simulink model "pfb_fir"  (Simulink 7.0)
settings: Solver=FixedStepDiscrete  SolverMode=SingleTasking  StartTime=0.0  StopTime=10.0  RelTol=1e-3
undefined symbols (not defined in the file): pfb_coefs
libraries: xbsIndex_r4 x385
(part 1 of 27)
settings Model: Creator=homin  LastModifiedBy=homin
settings DebuggingCC: SaveWithParameterizedLinksMsg=none  SignalResolutionControl=TryResolveAllWithWarning  MultiTaskDSMMsg=warning  MultiTaskCondExecSysMsg=none  StrictBusMsg=None
settings RTWCC: IncludeERTFirstTime=on
settings GRTTargetCC: TargetFcnLib=ansi_tfl_tmw.mat

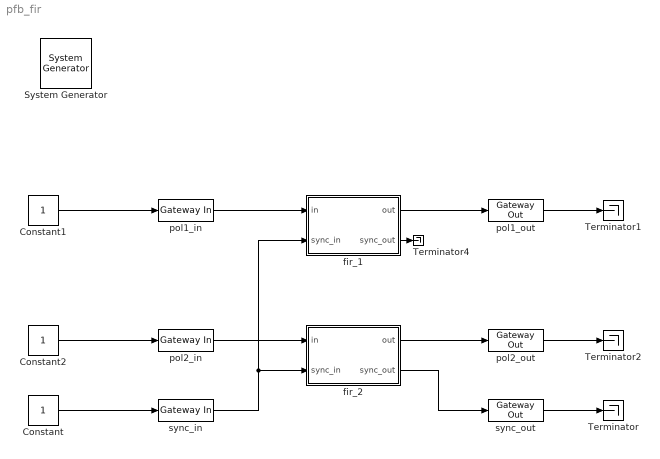
== system pfb_fir ==
  " System Generator" : xbsIndex_r4/ System Generator  Tag=genX  SystemSampleTime=-1  xilinxfamily=Virtex2P  part=xc2vp40  speed=-6  package=ff1152  synthesis_tool=XST  clock_wrapper=Clock Enables  directory=./pfb_fir_core  testbench=off  simulink_period=1  sysclk_period=100  dcm_input_clock_period=100  incr_netlist=off  trim_vbits=Everywhere in SubSystem  dbl_ovrd=According to Block Masks  core_generation=According to Block Masks  run_coregen=off  deprecated_control=off  eval_field=0  block_type=sysgen
      settings: block_version=10.1.3
  Constant : Constant  OutDataType=sfix(16)  OutScaling=2^0
  Constant1 : Constant  OutDataType=sfix(16)  OutScaling=2^0
  Constant2 : Constant  OutDataType=sfix(16)  OutScaling=2^0
  Terminator{,1..2,4} (4 alike) : Terminator
  fir_1 : Subsystem  AncestorBlock=newfft_library/FIR/fir  mask(FIR Filter){coefs=pfb_coefs(1024,6), n_bits_c=9, bin_pt_c=8, n_bits_d=8, bin_pt_d=7, n_bits_o=9, bin_pt_o=7, coef_bram=on, delay_bram=on, mult_latency=3, add_latency=1, show_sbo=on, munge_submasks=DumbDown}
      mask prompts: coefs "Tap Coefficients"; n_bits_c "Number of Coefficient Bits"; bin_pt_c "Coefficient Binary Point"; n_bits_d "Number of Data Bits"; bin_pt_d "Data Binary Point"; n_bits_o "Number of Bits Out"; bin_pt_o "Binary Point Out"; coef_bram "Use BRAM for Coefficients"; delay_bram "Use BRAM for Delay"; mult_latency "Multiplier Latency"; add_latency "Adder Latency"; show_sbo "Show Sub-Block Options"; munge_submasks "Sub-Block Masks"
      mask help: A Finite Impluse Response Filter. This FIR filter does not have provisions for folding the input sequence to improve multiplier efficiency, so it is suboptimal for "regular" (i.e. non-WOLA) FIR filters. It is intended primarily for WOLA (Weighted OverLap Add) FIR filters.
      mask init:
      | tic
      | fir_init(gcb, ...
      |   coefs, ...
      |   n_bits_c, ...
      |   bin_pt_c, ...
      |   n_bits_d, ...
      |   bin_pt_d, ...
      |   n_bits_o, ...
      |   bin_pt_o, ...
      |   coef_bram, ...
      |   delay_bram, ...
      |   mult_latency, ...
      |   add_latency, ...
      |   lower(get_param(gcb,'munge_submasks')) );
      | disp('fir_init complete.');
      | toc
      settings: AttributesFormatString=|
      | 6 taps
      | 9_8 coefs
      | 8_7 in
      | 9_7 out
      mask Help:
      | <pre>
      | Description::
      | 
      | A Finite Impluse Response Filter.
      | 
      | This Finite Impluse Response Filter does not have provisions for folding the input
      | sequence to improve multiplier efficiency, so it is suboptimal for "regular" (i.e. non-WOLA)
      | FIR filters.  It is intended primarily for WOLA (Weighted OverLap Add) FIR filters.
      | 
      | Mask Parameters::
      | 
      | Coefficiant(s) (coefs): Matrix of real double(s) to use as coefficient(s).
      | One column per tap.  Multiple rows will create a WOLA filter.
      | These should be specified as doubles.  They will be rounded/saturated according to the
      | specified number of bits (n_bits_c) and binary point (bin_pt_c).
      | 
      | Number of Coefficient Bits (n_bits_c): The number of bits used for the fixed point binary
      | representation of the coefficient(s).
      | 
      | Coefficient Binary Point (bin_pt_c): The binary point of the fixed point binary representation
      | of the coefficient(s).
      | 
      | Number of Data Bits (n_bits_d): The number of bits for real/imaginary components of the data.
      | 
      | Data Binary Point (bin_pt_d): The binary point for real/imaginary components of the data.
      | 
      | Number of Bits Out (n_bits_o): Specifies the width of the output (overflow wraps).
      | The internal adders will use a bit width of (n_bits_o-bin_pt_o+bin_pt_c+bin_pt_d).
      | 
      | Binary Point Out (bin_pt_o): Specifies the binary point of the output (quantization truncates).
      | The internal adders will use a binary point of (bin_pt_c+bin_pt_d).
      | 
      | Use BRAM for Coefficients (coef_bram): Check this checkbox to store the coefficients in BRAM.
      | If unchecked, the coefficients will be stored in distributed memory (i.e. slices).
      | This is only relevant is length(coef) is greater than 1; otherwise, a constant block is used.
      | 
      | Use BRAM for Delay (delay_bram): Check this checkbox to implement the delay using BRAM.
      | If unchecked, the delay will be implemented using SLR16 elements (i.e. slices).
      | 
      | Multiplier Latency (mult_latency): Latency to use for the underlying multiplier.
      | 
      | Adder Latency (add_latency): Latency to use for the underlying adder.
      | </pre>
      mask StyleString: edit,edit,edit,edit,edit,edit,edit,checkbox,checkbox,edit,edit,checkbox,popup(Keep|DumbDown|Unmask)
      mask CallbackString:
      | |||||||||||mvs=get_param(gcb,'MaskVisibilityString');
      | if strcmp(get_param(gcb,'show_sbo'),'on')
      |   onoff='on';
      | else
      |   onoff='off';
      | end
      | mvs=regexprep(mvs,'o[nf]*$',onoff);
      | set_param(gcb,'MaskVisibilityString',mvs);
      | |
  fir_2 : Subsystem  AncestorBlock=newfft_library/FIR/fir  mask(FIR Filter){coefs=pfb_coefs(1024,6), n_bits_c=9, bin_pt_c=8, n_bits_d=8, bin_pt_d=7, n_bits_o=9, bin_pt_o=7, coef_bram=on, delay_bram=on, mult_latency=3, add_latency=1, show_sbo=on, munge_submasks=DumbDown}
      mask prompts: coefs "Tap Coefficients"; n_bits_c "Number of Coefficient Bits"; bin_pt_c "Coefficient Binary Point"; n_bits_d "Number of Data Bits"; bin_pt_d "Data Binary Point"; n_bits_o "Number of Bits Out"; bin_pt_o "Binary Point Out"; coef_bram "Use BRAM for Coefficients"; delay_bram "Use BRAM for Delay"; mult_latency "Multiplier Latency"; add_latency "Adder Latency"; show_sbo "Show Sub-Block Options"; munge_submasks "Sub-Block Masks"
      mask help: A Finite Impluse Response Filter. This FIR filter does not have provisions for folding the input sequence to improve multiplier efficiency, so it is suboptimal for "regular" (i.e. non-WOLA) FIR filters. It is intended primarily for WOLA (Weighted OverLap Add) FIR filters.
      mask init: same as pfb_fir/fir_1
      settings: AttributesFormatString=|
      | 6 taps
      | 9_8 coefs
      | 8_7 in
      | 9_7 out
      mask Help:
      | <pre>
      | Description::
      | 
      | A Finite Impluse Response Filter.
      | 
      | This Finite Impluse Response Filter does not have provisions for folding the input
      | sequence to improve multiplier efficiency, so it is suboptimal for "regular" (i.e. non-WOLA)
      | FIR filters.  It is intended primarily for WOLA (Weighted OverLap Add) FIR filters.
      | 
      | Mask Parameters::
      | 
      | Coefficiant(s) (coefs): Matrix of real double(s) to use as coefficient(s).
      | One column per tap.  Multiple rows will create a WOLA filter.
      | These should be specified as doubles.  They will be rounded/saturated according to the
      | specified number of bits (n_bits_c) and binary point (bin_pt_c).
      | 
      | Number of Coefficient Bits (n_bits_c): The number of bits used for the fixed point binary
      | representation of the coefficient(s).
      | 
      | Coefficient Binary Point (bin_pt_c): The binary point of the fixed point binary representation
      | of the coefficient(s).
      | 
      | Number of Data Bits (n_bits_d): The number of bits for real/imaginary components of the data.
      | 
      | Data Binary Point (bin_pt_d): The binary point for real/imaginary components of the data.
      | 
      | Number of Bits Out (n_bits_o): Specifies the width of the output (overflow wraps).
      | The internal adders will use a bit width of (n_bits_o-bin_pt_o+bin_pt_c+bin_pt_d).
      | 
      | Binary Point Out (bin_pt_o): Specifies the binary point of the output (quantization truncates).
      | The internal adders will use a binary point of (bin_pt_c+bin_pt_d).
      | 
      | Use BRAM for Coefficients (coef_bram): Check this checkbox to store the coefficients in BRAM.
      | If unchecked, the coefficients will be stored in distributed memory (i.e. slices).
      | This is only relevant is length(coef) is greater than 1; otherwise, a constant block is used.
      | 
      | Use BRAM for Delay (delay_bram): Check this checkbox to implement the delay using BRAM.
      | If unchecked, the delay will be implemented using SLR16 elements (i.e. slices).
      | 
      | Multiplier Latency (mult_latency): Latency to use for the underlying multiplier.
      | 
      | Adder Latency (add_latency): Latency to use for the underlying adder.
      | </pre>
      mask StyleString: edit,edit,edit,edit,edit,edit,edit,checkbox,checkbox,edit,edit,checkbox,popup(Keep|DumbDown|Unmask)
      mask CallbackString:
      | |||||||||||mvs=get_param(gcb,'MaskVisibilityString');
      | if strcmp(get_param(gcb,'show_sbo'),'on')
      |   onoff='on';
      | else
      |   onoff='off';
      | end
      | mvs=regexprep(mvs,'o[nf]*$',onoff);
      | set_param(gcb,'MaskVisibilityString',mvs);
      | |
  pol1_in : xbsIndex_r4/Gateway In  arith_type=Unsigned  n_bits=16  bin_pt=0  quantization=Truncate  overflow=Wrap  period=1  dbl_ovrd=off  timing_constraint=None  locs_specified=off  LOCs={}  block_type=gatewayin
      settings: infoedit="Gateway in block.  Converts inputs of type Simulink integer, double and fixed point to  Xilinx fixed point type.<P><P>Hardware notes:  In hardware these blocks become top level input ports."  xl_area=[0, 0, 0, 0, 0, 0, 0]  block_version=10.1.3
  pol1_out : xbsIndex_r4/Gateway Out  hdl_port=on  timing_constraint=None  locs_specified=off  LOCs={}  block_type=gatewayout
      settings: infoedit="Gateway out block.  Converts Xilinx fixed point inputs into ouputs of type Simulink integer, double, or fixed point.<P><P>Hardware notes:  In hardware these blocks become top level output ports or are discarded, depending on how they are configured."  xl_area=[0, 0, 0, 0, 0, 0, 0]  block_version=10.1.3
  pol2_in : xbsIndex_r4/Gateway In  arith_type=Unsigned  n_bits=16  bin_pt=0  quantization=Truncate  overflow=Wrap  period=1  dbl_ovrd=off  timing_constraint=None  locs_specified=off  LOCs={}  block_type=gatewayin
      settings: infoedit="Gateway in block.  Converts inputs of type Simulink integer, double and fixed point to  Xilinx fixed point type.<P><P>Hardware notes:  In hardware these blocks become top level input ports."  xl_area=[0, 0, 0, 0, 0, 0, 0]  block_version=10.1.3
  pol2_out : xbsIndex_r4/Gateway Out  hdl_port=on  timing_constraint=None  locs_specified=off  LOCs={}  block_type=gatewayout
      settings: infoedit="Gateway out block.  Converts Xilinx fixed point inputs into ouputs of type Simulink integer, double, or fixed point.<P><P>Hardware notes:  In hardware these blocks become top level output ports or are discarded, depending on how they are configured."  xl_area=[0, 0, 0, 0, 0, 0, 0]  block_version=10.1.3
  sync_in : xbsIndex_r4/Gateway In  arith_type=Boolean  n_bits=8  bin_pt=6  quantization=Truncate  overflow=Wrap  period=1  dbl_ovrd=off  timing_constraint=None  locs_specified=off  LOCs={}  block_type=gatewayin
      settings: infoedit="Gateway in block.  Converts inputs of type Simulink integer, double and fixed point to  Xilinx fixed point type.<P><P>Hardware notes:  In hardware these blocks become top level input ports."  xl_area=[0, 0, 0, 0, 0, 0, 0]  block_version=10.1.3
  sync_out : xbsIndex_r4/Gateway Out  hdl_port=on  timing_constraint=None  locs_specified=off  LOCs={}  block_type=gatewayout
      settings: infoedit="Gateway out block.  Converts Xilinx fixed point inputs into ouputs of type Simulink integer, double, or fixed point.<P><P>Hardware notes:  In hardware these blocks become top level output ports or are discarded, depending on how they are configured."  xl_area=[0, 0, 0, 0, 0, 0, 0]  block_version=10.1.3
  wires:
  sync_in/1 -> fir_2/2(sync_in), fir_1/2(sync_in)
  Constant/1 -> sync_in/1
  Constant1/1 -> pol1_in/1
  sync_out/1 -> Terminator/1
  pol1_out/1 -> Terminator1/1
  pol1_in/1 -> fir_1/1(in)
  fir_1/1(out) -> pol1_out/1
  Constant2/1 -> pol2_in/1
  pol2_in/1 -> fir_2/1(in)
  pol2_out/1 -> Terminator2/1
  fir_2/1(out) -> pol2_out/1
  fir_2/2(sync_out) -> sync_out/1
  fir_1/2(sync_out) -> Terminator4/1
